simulink model "Zero_6C_5000"  (R2019a)
settings: Solver=VariableStepAuto  StartTime=0.0  StopTime=100000  RelTol=1e-3
libraries: fl_lib x40, nesl_utility x14, ee_lib x8, SimscapeFluids_lib x2, simulink x1
settings Model: Creator=Abd  LastModifiedBy=User

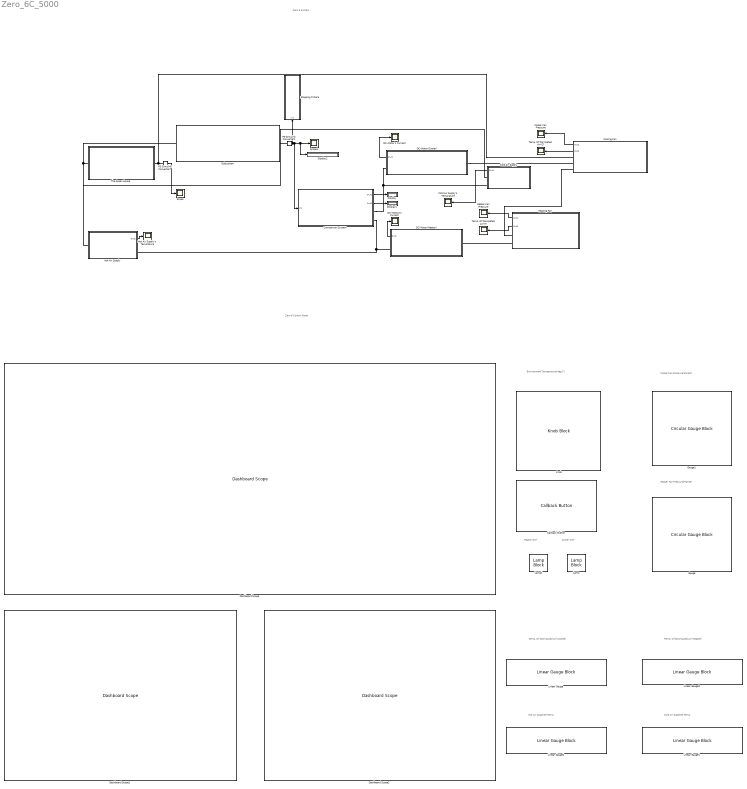
== system Zero_6C_5000 ==
  note: Environment Temperature(deg C)
  note: Temp. Of Distriputed Air(Cooled)
  note: Zero 6 System
  note: Heater ON?
  note: Cooler ON?
  note: Cooler Fan Pressure(Pa*e3)
  note: Heater Fan Pressure(Pa*e3)
  note: Temp. Of Distriputed Air(Heated)
  note: Hot Air Supplied Temp.
  note: Cold Air Supplied Temp.
  note: Zero 6 Control Panel
  Callback Button : CallbackButton  ButtonText=Start Simulation
      settings: ClickFcn=|
      | % name of your model
      | modelName = 'Zero_6C_5000';
      | 
      | % sim will simulate the model in argument
      | sim(modelName);
  Cold Air Supply : Subsystem
  Cold Air Supply's Temprature : Scope
  Comparison System : Subsystem
  Cooler Fan Pressure : Scope
  Cooling Fan : Subsystem
  DC-Motor's Current : Scope
  DC-Motor(Cooler) : Subsystem
  DC-Motor(Heater) : Subsystem
  DC-Motor2's Current : Scope
  Dashboard Scope : DashboardScope  Ymin=-20  Ymax=60
  Dashboard Scope1 : DashboardScope  ShowInitialText=off  TimeSpan=3  Ymin=-1  Ymax=4
  Dashboard Scope2 : DashboardScope  Ymin=0  Ymax=10
  Display : Display
  Display1 : Display
  Display2 : Display
      settings: Format=long_e
  Gauge : CircularGaugeBlock  LabelPosition=Hide  ScaleMin=60  ScaleMax=101.5
  Gauge1 : CircularGaugeBlock  LabelPosition=Hide  ScaleMin=60  ScaleMax=101.5
  Heater Fan Pressure : Scope
  Heating Fan : Subsystem
  Hot Air Supply : Subsystem
  Hot Air Supply's Temprature : Scope
  Knob : KnobBlock  LabelPosition=Hide  ScaleMin=-20  ScaleMax=60
  Lamp : LampBlock  LabelPosition=Hide
  Lamp1 : LampBlock  LabelPosition=Hide
  Linear Gauge{,1..3} (4 alike) : LinearGaugeBlock  LabelPosition=Hide  ScaleMin=-20  ScaleMax=60
  PS-Simulink Converter1 : nesl_utility/PS-Simulink Converter  PhysicalDomain=network_engine_domain  SubClassName=ps_output  LeftPortType=input  RightPortType=output  PseudoPeriodic=off  Frequencies=[]  Unit=1  AffineConversion=off
  PS-Simulink Converter7 : nesl_utility/PS-Simulink Converter  PhysicalDomain=network_engine_domain  SubClassName=ps_output  LeftPortType=input  RightPortType=output  PseudoPeriodic=off  Frequencies=[]  Unit=1  AffineConversion=off
  Scope : Scope
  Scope1 : Scope
  Stopping Critera : Subsystem
  Subsystem : Subsystem
  Temp. Of Dissipated Air(C) : Scope
  Temp. Of Dissipated Air(H) : Scope
  The Green House : Subsystem
  wires:
  PS-Simulink Converter1/1 -> Comparison System/1(In1), Display2/1, Scope1/1, Stopping Critera/1(In1)
  DC-Motor(Cooler)/1(Out1) -> DC-Motor's Current/1
  Cooling Fan/1(Out1) -> Cooler Fan Pressure/1
  Cooling Fan/2(Out2) -> Temp. Of Dissipated Air(C)/1
  Heating Fan/1(Out1) -> Heater Fan Pressure/1
  Heating Fan/2(Out2) -> Temp. Of Dissipated Air(H)/1
  DC-Motor(Heater)/1(Out1) -> DC-Motor2's Current/1
  Cold Air Supply/1(Out1) -> Cold Air Supply's Temprature/1
  Hot Air Supply/1(Out1) -> Hot Air Supply's Temprature/1
  PS-Simulink Converter7/1 -> Scope/1
  Comparison System/2(Out2) -> Display1/1
  Comparison System/1(Out1) -> Display/1
  connections:
  PS-Simulink Converter7/LConn1 -- Cooling Fan/RConn1 -- The Green House/RConn1
  The Green House/LConn1 -- Subsystem/LConn1 -- Cold Air Supply/RConn1 -- Hot Air Supply/LConn1
  DC-Motor(Cooler)/LConn1 -- Cooling Fan/RConn2
  Cooling Fan/RConn3 -- Heating Fan/RConn1
  Heating Fan/RConn2 -- DC-Motor(Heater)/LConn1
  Comparison System/RConn1 -- Cold Air Supply/RConn2 -- DC-Motor(Cooler)/RConn1
  Comparison System/RConn2 -- Hot Air Supply/RConn1 -- DC-Motor(Heater)/RConn1
  PS-Simulink Converter1/LConn1 -- Subsystem/RConn1

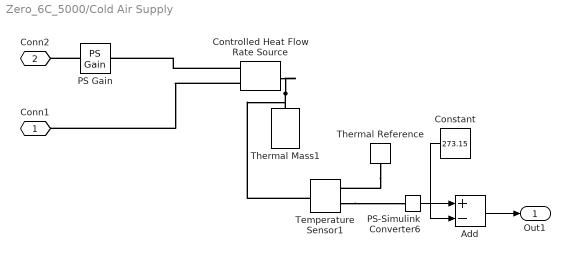
== system Zero_6C_5000/Cold Air Supply ==
  Add : Sum  Inputs=+-
  Constant : Constant  Value=273.15
  Controlled Heat Flow Rate Source : fl_lib/Thermal/Thermal Sources/Controlled Heat Flow Rate Source
      settings: SourceProductName=Simscape
  PS Gain : fl_lib/Physical Signals/Functions/PS Gain  gain=10
  PS-Simulink Converter6 : nesl_utility/PS-Simulink Converter  PhysicalDomain=network_engine_domain  SubClassName=ps_output  LeftPortType=input  RightPortType=output  PseudoPeriodic=off  Frequencies=[]  Unit=1  AffineConversion=off
  Temperature Sensor1 : fl_lib/Thermal/Thermal Sensors/Temperature Sensor
  Thermal Mass1 : fl_lib/Thermal/Thermal Elements/Thermal Mass  mass=100 kg  sp_heat=1.0045e3 J/kg/K  T_specify=on  T_priority=High  T=273.15 K  T_nominal_specify=off  T_nominal_unit=K  T_nominal_value=1  Q_specify=off  Q_priority=None  Q=0 W  Q_nominal_specify=off  Q_nominal_unit=W  Q_nominal_value=1
  Thermal Reference : fl_lib/Thermal/Thermal Elements/Thermal Reference
  Conn1 : PMIOPort  Side=Right
  Conn2 : PMIOPort  Port=2  Side=Right
  Out1 : Outport
  wires:
  Constant/1 -> Add/2
  Add/1 -> Out1/1
  PS-Simulink Converter6/1 -> Add/1
  connections:
  Temperature Sensor1/RConn2 -- PS-Simulink Converter6/LConn1
  Thermal Reference/LConn1 -- Temperature Sensor1/RConn1
  PS Gain/LConn1 -- Conn2/RConn1
  Controlled Heat Flow Rate Source/RConn2 -- Conn1/RConn1
  Thermal Mass1/LConn1 -- Controlled Heat Flow Rate Source/LConn1 -- Temperature Sensor1/LConn1
  Controlled Heat Flow Rate Source/RConn1 -- PS Gain/RConn1

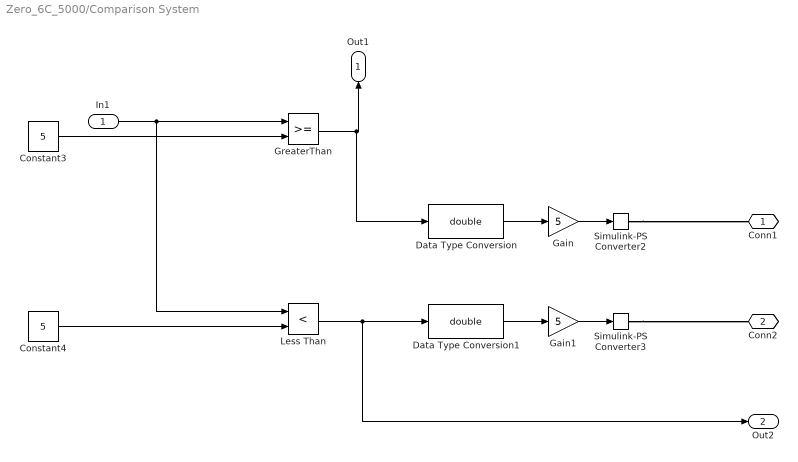
== system Zero_6C_5000/Comparison System ==
  In1 : Inport
  Constant3 : Constant  Value=5
  Constant4 : Constant  Value=5
  Data Type Conversion : DataTypeConversion  OutDataTypeStr=double
  Data Type Conversion1 : DataTypeConversion  OutDataTypeStr=double
  Gain : Gain  Gain=5
  Gain1 : Gain  Gain=5
  GreaterThan : RelationalOperator  OutDataTypeStr=boolean  RndMeth=Simplest
  Less Than : RelationalOperator  Operator=<  OutDataTypeStr=boolean  RndMeth=Simplest
  Simulink-PS Converter2 : nesl_utility/Simulink-PS Converter  PhysicalDomain=network_engine_domain  SubClassName=ps_input  LeftPortType=input  RightPortType=output  PseudoPeriodic=off  Frequencies=[]  NoiseDistribution=none  NoiseParameters=[]  Unit=1  AffineConversion=off  FilteringAndDerivatives=provide  SimscapeFilterOrder=1  InputFilterTimeConstant=0.001  UdotUserProvided=0
  Simulink-PS Converter3 : nesl_utility/Simulink-PS Converter  PhysicalDomain=network_engine_domain  SubClassName=ps_input  LeftPortType=input  RightPortType=output  PseudoPeriodic=off  Frequencies=[]  NoiseDistribution=none  NoiseParameters=[]  Unit=1  AffineConversion=off  FilteringAndDerivatives=provide  SimscapeFilterOrder=1  InputFilterTimeConstant=0.001  UdotUserProvided=0
  Conn1 : PMIOPort  Side=Right
  Conn2 : PMIOPort  Port=2  Side=Right
  Out1 : Outport
  Out2 : Outport  Port=2
  wires:
  Less Than/1 -> Out2/1, Data Type Conversion1/1
  Gain/1 -> Simulink-PS Converter2/1
  Data Type Conversion/1 -> Gain/1
  Constant3/1 -> GreaterThan/2
  Gain1/1 -> Simulink-PS Converter3/1
  GreaterThan/1 -> Data Type Conversion/1, Out1/1
  Constant4/1 -> Less Than/2
  Data Type Conversion1/1 -> Gain1/1
  In1/1 -> GreaterThan/1, Less Than/1
  connections:
  Simulink-PS Converter3/RConn1 -- Conn2/RConn1
  Simulink-PS Converter2/RConn1 -- Conn1/RConn1

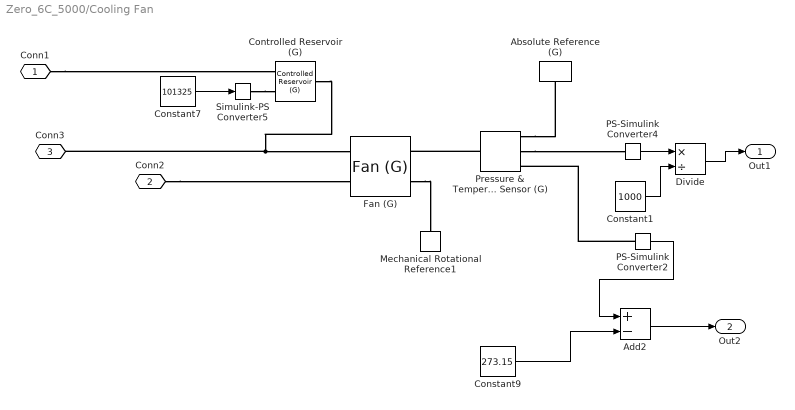
== system Zero_6C_5000/Cooling Fan ==
  Absolute Reference (G) : fl_lib/Gas/Elements/Absolute Reference (G)
      settings: SourceProductName=Simscape  SourceProductBaseCode=SS
  Add2 : Sum  Inputs=+-
  Constant1 : Constant  Value=1000
  Constant7 : Constant  Value=101325
  Constant9 : Constant  Value=273.15
  Controlled Reservoir (G) : fl_lib/Gas/Elements/Controlled Reservoir (G)  area_A=0.01 m^2
      settings: SourceProductName=Simscape  SourceProductBaseCode=SS
  Divide : Product  Inputs=*/
  Fan (G) : SimscapeFluids_lib/Gas/Turbomachinery/Fan (G)  fan_spec=fluids.gas.enum.fan_spec.table1D  mech_orientation=simscape.enum.posneg.positive  flow_rate_1D_TLU=[4.7, 5.2, 5.7, 6.1, 6.6] m^3/s  Dp_1D_TLU=[1120, 995.36, 870.94, 746.52, 622.1] Pa  eta_1D_TLU=[.1, .2, .25, .15, .1]  rho_ref_1D=1.2 kg/m^3  omega_ref_1D=910 rpm  omega_Dp_TLU=[450, 500, 550, 600, 650] rpm  flow_rate_Dp_TLU=[.2, .3, .4, .5] m^3/s  Dp_TLU=[675, 650, 560, 420; 830, 800, 695, 520; 1008, 966, 840, 630; 1200, 1150, 1000, 750; 1370, 1300, 1250, 1000] Pa  eta_Dp_TLU=[.22, .23, .25, .24; .38, .39, .4, .34; .58, .6, .62, .6; .81, .82, .84, .8; .88, .91, .95, .9]  omega_flow_TLU=[1800, 2000, 2400, 2800, 3000] rpm  Dp_flow_TLU=[1 / 8, 1 / 4, 3 / 8, 1 / 2] * 3386.4 Pa  flow_rate_TLU=[.3282, .2965, .2556, .1973; .8254, .71, .5876, .4545; 1.2018, 1.0829, .9083, .7034; 1.5065, 1.4098, 1.2722, .9844; 1.8368, 1.7507, 1.6055, 1.2417] m^3/s  eta_flow_TLU=[.22, .23, .25, .24; .38, .39, .4, .34; .58, .6, .62, .6; .81, .82, .84, .8; .88, .91, .95, .9]  omega_DpMax_TLU=[1800, 2000, 2400, 2800, 3000] rpm  DpMax_TLU=[1 / 8, 1 / 4, 3 / 8, 1 / 2, 5 / 8] * 3386.4 Pa  omega_flow_TLU_=[1800, 2000, 2400, 2800, 3000] rpm  Dp_DpMax_TLU=linspace(0, 1, 7)  flow_rate_TLU_=[.3282, .2965, .2556, .1973, .1799, .1288, .0736; .8254, .71, .5876, .4545, .4157, .2967, .1696; 1.2018, 1.0829, .9083, .7034, .6415, .4584, .2619; 1.5065, 1.4098, 1.2722, .9844, .8991, .6418, .3668; 1.8368, 1.7507, 1.6055, 1.2417, 1.1337, .8098, .464] m^3/s  eta_flow_TLU_=[.22, .23, .25, .26, .27, .275, .28; .38, .39, .4, .41, .42, .425, .43; .48, .5, .52, .54, .55, .54, .53; .4, .42, .44, .46, .48, .45, .44; .42, .43, .45, .47, .49, .46, .44]  rho_ref_2D=1.2 kg/m^3  omega_threshold=1 rpm  area_A=0.01 m^2  area_B=0.01 m^2
      settings: SourceProductName=Simscape Fluids  SourceProductBaseCode=SH
  Mechanical Rotational Reference1 : fl_lib/Mechanical/Rotational Elements/Mechanical Rotational Reference
  PS-Simulink Converter2 : nesl_utility/PS-Simulink Converter  PhysicalDomain=network_engine_domain  SubClassName=ps_output  LeftPortType=input  RightPortType=output  PseudoPeriodic=off  Frequencies=[]  Unit=1  AffineConversion=off
  PS-Simulink Converter4 : nesl_utility/PS-Simulink Converter  PhysicalDomain=network_engine_domain  SubClassName=ps_output  LeftPortType=input  RightPortType=output  PseudoPeriodic=off  Frequencies=[]  Unit=1  AffineConversion=off
  Pressure & Temperature Sensor (G) : fl_lib/Gas/Sensors/Pressure & Temperature Sensor (G)
      settings: SourceProductName=Simscape  SourceProductBaseCode=SS
  Simulink-PS Converter5 : nesl_utility/Simulink-PS Converter  PhysicalDomain=network_engine_domain  SubClassName=ps_input  LeftPortType=input  RightPortType=output  PseudoPeriodic=off  Frequencies=[]  NoiseDistribution=none  NoiseParameters=[]  Unit=1  AffineConversion=off  FilteringAndDerivatives=provide  SimscapeFilterOrder=1  InputFilterTimeConstant=0.001  UdotUserProvided=0
  Conn1 : PMIOPort  Side=Right
  Conn2 : PMIOPort  Port=2  Side=Right
  Conn3 : PMIOPort  Port=3  Side=Right
  Out1 : Outport
  Out2 : Outport  Port=2
  wires:
  Constant9/1 -> Add2/2
  Constant7/1 -> Simulink-PS Converter5/1
  PS-Simulink Converter2/1 -> Add2/1
  Add2/1 -> Out2/1
  Divide/1 -> Out1/1
  PS-Simulink Converter4/1 -> Divide/1
  Constant1/1 -> Divide/2
  connections:
  Controlled Reservoir (G)/LConn1 -- Fan (G)/RConn1 -- Conn3/RConn1
  Pressure & Temperature Sensor (G)/RConn2 -- PS-Simulink Converter4/LConn1
  PS-Simulink Converter2/LConn1 -- Pressure & Temperature Sensor (G)/RConn3
  Pressure & Temperature Sensor (G)/RConn1 -- Absolute Reference (G)/LConn1
  Simulink-PS Converter5/RConn1 -- Controlled Reservoir (G)/RConn2
  Conn1/RConn1 -- Controlled Reservoir (G)/RConn1
  Pressure & Temperature Sensor (G)/LConn1 -- Fan (G)/LConn1
  Fan (G)/LConn2 -- Mechanical Rotational Reference1/LConn1
  Conn2/RConn1 -- Fan (G)/RConn2

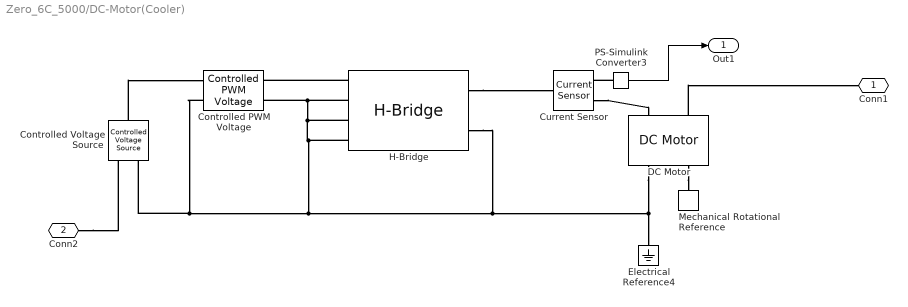
== system Zero_6C_5000/DC-Motor(Cooler) ==
  Controlled PWM Voltage : ee_lib/Integrated Circuits/Controlled PWM Voltage  F=4000 Hz  TD=0 s  pulse_width_offset=0 s  pulse_min=0 s  Vmin=0 V  Vmax=5 V  Vm=5 V  pwm_or_av=2  event_type=1  sample_time=1e-6 s  u_min=0  u_max=1
      settings: SourceProductName=Simscape Electrical
  Controlled Voltage Source : fl_lib/Electrical/Electrical Sources/Controlled Voltage Source
  Current Sensor : fl_lib/Electrical/Electrical Sensors/Current Sensor
  DC Motor : ee_lib/Electromechanical/Brushed Motors/DC Motor  parameterization=3  Ra=3.9 Ohm  La=0.01 H  emf_or_torque=1  Kv=0.072e-3 V/rpm  Ki=6.876e-4 N*m/A  T_stall=0.24e-3 N*m  w_max=4000 rpm  w_rated=2500 rpm  P_rated=10 W  V_rated=12 V  J=2000 g*cm^2  lam_param=1  lam=1e-6 N*m/(rad/s)  i_noload=0 A  V_i_noload=1.5 V  speed0=0 rpm  alpha=3.93e-3 1/K  Tmeas=25 degC  thermal_mass=100 J/K  initial_temperature=25 degC
      settings: SourceProductName=Simscape Electrical
  Electrical Reference4 : fl_lib/Electrical/Electrical Elements/Electrical Reference
  H-Bridge : ee_lib/Semiconductors & Converters/Converters/H-Bridge  Venable=2.5 V  Vmax=5.0 V  Vreverse=2.5 V  Vbrake=2.5 V  Vm=12 V  pwm_or_av=2  discontinuous=0  freewheeling_mode=1  freewheeling_mode_disc=1  Ron=0.1 Ohm  Don=0.05 Ohm  Rload=10 Ohm  Lload=1e-5 H  F=10 kHz  thermal_mass=100 J/K  initial_temperature=298.15 K  Ron2=0.1 Ohm  Don2=0.05 Ohm  Tmeas=298.15 K  Tmeas2=398.15 K
      settings: SourceProductName=Simscape Electrical
  Mechanical Rotational Reference : fl_lib/Mechanical/Rotational Elements/Mechanical Rotational Reference
  PS-Simulink Converter3 : nesl_utility/PS-Simulink Converter  PhysicalDomain=network_engine_domain  SubClassName=ps_output  LeftPortType=input  RightPortType=output  PseudoPeriodic=off  Frequencies=[]  Unit=1  AffineConversion=off
  Conn1 : PMIOPort  Side=Left
  Conn2 : PMIOPort  Port=2  Side=Right
  Out1 : Outport
  wires:
  PS-Simulink Converter3/1 -> Out1/1
  connections:
  H-Bridge/LConn3 -- Electrical Reference4/LConn1 -- DC Motor/RConn1 -- H-Bridge/RConn2 -- Controlled Voltage Source/RConn2 -- Controlled PWM Voltage/LConn2 -- H-Bridge/LConn4 -- H-Bridge/LConn2 -- Controlled PWM Voltage/RConn2
  Controlled Voltage Source/LConn1 -- Controlled PWM Voltage/LConn1
  DC Motor/RConn2 -- Mechanical Rotational Reference/LConn1
  DC Motor/LConn2 -- Conn1/RConn1
  H-Bridge/LConn1 -- Controlled PWM Voltage/RConn1
  PS-Simulink Converter3/LConn1 -- Current Sensor/RConn1
  Current Sensor/RConn2 -- DC Motor/LConn1
  H-Bridge/RConn1 -- Current Sensor/LConn1
  Conn2/RConn1 -- Controlled Voltage Source/RConn1

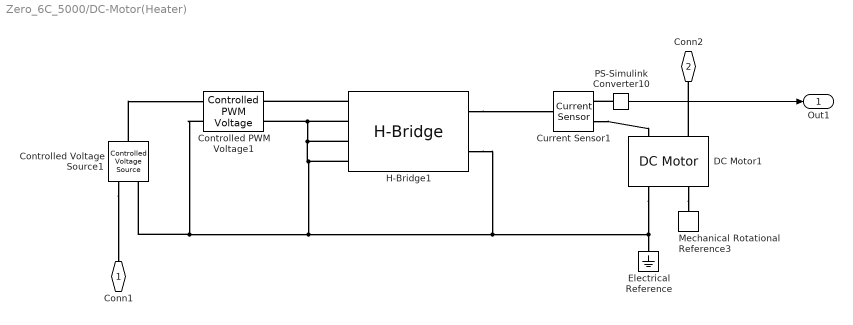
== system Zero_6C_5000/DC-Motor(Heater) ==
  Controlled PWM Voltage1 : ee_lib/Integrated Circuits/Controlled PWM Voltage  F=4000 Hz  TD=0 s  pulse_width_offset=0 s  pulse_min=0 s  Vmin=0 V  Vmax=5 V  Vm=5 V  pwm_or_av=2  event_type=1  sample_time=1e-6 s  u_min=0  u_max=1
      settings: SourceProductName=Simscape Electrical
  Controlled Voltage Source1 : fl_lib/Electrical/Electrical Sources/Controlled Voltage Source
  Current Sensor1 : fl_lib/Electrical/Electrical Sensors/Current Sensor
  DC Motor1 : ee_lib/Electromechanical/Brushed Motors/DC Motor  parameterization=3  Ra=3.9 Ohm  La=0.01 H  emf_or_torque=1  Kv=0.072e-3 V/rpm  Ki=6.876e-4 N*m/A  T_stall=0.24e-3 N*m  w_max=4000 rpm  w_rated=2500 rpm  P_rated=10 W  V_rated=12 V  J=2000 g*cm^2  lam_param=1  lam=1e-6 N*m/(rad/s)  i_noload=0 A  V_i_noload=1.5 V  speed0=0 rpm  alpha=3.93e-3 1/K  Tmeas=25 degC  thermal_mass=100 J/K  initial_temperature=25 degC
      settings: SourceProductName=Simscape Electrical
  Electrical Reference : fl_lib/Electrical/Electrical Elements/Electrical Reference
  H-Bridge1 : ee_lib/Semiconductors & Converters/Converters/H-Bridge  Venable=2.5 V  Vmax=5.0 V  Vreverse=2.5 V  Vbrake=2.5 V  Vm=12 V  pwm_or_av=2  discontinuous=0  freewheeling_mode=1  freewheeling_mode_disc=1  Ron=0.1 Ohm  Don=0.05 Ohm  Rload=10 Ohm  Lload=1e-5 H  F=10 kHz  thermal_mass=100 J/K  initial_temperature=298.15 K  Ron2=0.1 Ohm  Don2=0.05 Ohm  Tmeas=298.15 K  Tmeas2=398.15 K
      settings: SourceProductName=Simscape Electrical
  Mechanical Rotational Reference3 : fl_lib/Mechanical/Rotational Elements/Mechanical Rotational Reference
  PS-Simulink Converter10 : nesl_utility/PS-Simulink Converter  PhysicalDomain=network_engine_domain  SubClassName=ps_output  LeftPortType=input  RightPortType=output  PseudoPeriodic=off  Frequencies=[]  Unit=1  AffineConversion=off
  Conn1 : PMIOPort  Side=Right
  Conn2 : PMIOPort  Port=2  Side=Left
  Out1 : Outport
  wires:
  PS-Simulink Converter10/1 -> Out1/1
  connections:
  Controlled Voltage Source1/RConn1 -- Conn1/RConn1
  PS-Simulink Converter10/LConn1 -- Current Sensor1/RConn1
  H-Bridge1/LConn3 -- Controlled PWM Voltage1/RConn2 -- H-Bridge1/LConn2 -- H-Bridge1/LConn4 -- Controlled PWM Voltage1/LConn2 -- Controlled Voltage Source1/RConn2 -- H-Bridge1/RConn2 -- Electrical Reference/LConn1 -- DC Motor1/RConn1
  Controlled Voltage Source1/LConn1 -- Controlled PWM Voltage1/LConn1
  Current Sensor1/RConn2 -- DC Motor1/LConn1
  DC Motor1/RConn2 -- Mechanical Rotational Reference3/LConn1
  H-Bridge1/RConn1 -- Current Sensor1/LConn1
  H-Bridge1/LConn1 -- Controlled PWM Voltage1/RConn1
  DC Motor1/LConn2 -- Conn2/RConn1

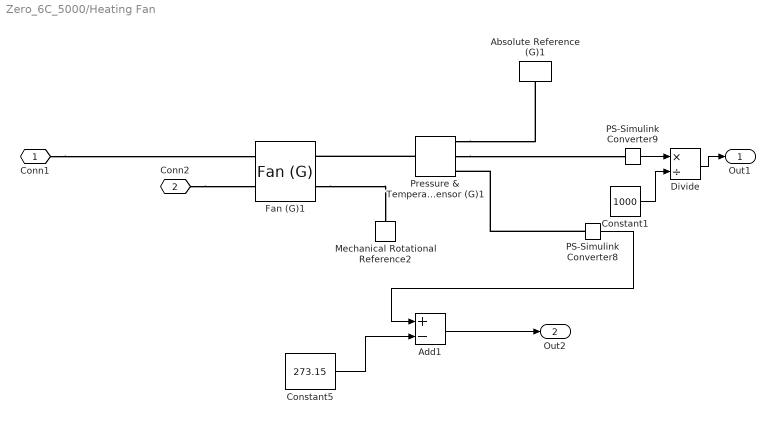
== system Zero_6C_5000/Heating Fan ==
  Absolute Reference (G)1 : fl_lib/Gas/Elements/Absolute Reference (G)
      settings: SourceProductName=Simscape  SourceProductBaseCode=SS
  Add1 : Sum  Inputs=+-
  Constant1 : Constant  Value=1000
  Constant5 : Constant  Value=273.15
  Divide : Product  Inputs=*/
  Fan (G)1 : SimscapeFluids_lib/Gas/Turbomachinery/Fan (G)  fan_spec=fluids.gas.enum.fan_spec.table1D  mech_orientation=simscape.enum.posneg.positive  flow_rate_1D_TLU=[4.7, 5.2, 5.7, 6.1, 6.6] m^3/s  Dp_1D_TLU=[1120, 995.36, 870.94, 746.52, 622.1] Pa  eta_1D_TLU=[.1, .2, .25, .15, .1]  rho_ref_1D=1.2 kg/m^3  omega_ref_1D=910 rpm  omega_Dp_TLU=[450, 500, 550, 600, 650] rpm  flow_rate_Dp_TLU=[.2, .3, .4, .5] m^3/s  Dp_TLU=[675, 650, 560, 420; 830, 800, 695, 520; 1008, 966, 840, 630; 1200, 1150, 1000, 750; 1370, 1300, 1250, 1000] Pa  eta_Dp_TLU=[.22, .23, .25, .24; .38, .39, .4, .34; .58, .6, .62, .6; .81, .82, .84, .8; .88, .91, .95, .9]  omega_flow_TLU=[1800, 2000, 2400, 2800, 3000] rpm  Dp_flow_TLU=[1 / 8, 1 / 4, 3 / 8, 1 / 2] * 3386.4 Pa  flow_rate_TLU=[.3282, .2965, .2556, .1973; .8254, .71, .5876, .4545; 1.2018, 1.0829, .9083, .7034; 1.5065, 1.4098, 1.2722, .9844; 1.8368, 1.7507, 1.6055, 1.2417] m^3/s  eta_flow_TLU=[.22, .23, .25, .24; .38, .39, .4, .34; .58, .6, .62, .6; .81, .82, .84, .8; .88, .91, .95, .9]  omega_DpMax_TLU=[1800, 2000, 2400, 2800, 3000] rpm  DpMax_TLU=[1 / 8, 1 / 4, 3 / 8, 1 / 2, 5 / 8] * 3386.4 Pa  omega_flow_TLU_=[1800, 2000, 2400, 2800, 3000] rpm  Dp_DpMax_TLU=linspace(0, 1, 7)  flow_rate_TLU_=[.3282, .2965, .2556, .1973, .1799, .1288, .0736; .8254, .71, .5876, .4545, .4157, .2967, .1696; 1.2018, 1.0829, .9083, .7034, .6415, .4584, .2619; 1.5065, 1.4098, 1.2722, .9844, .8991, .6418, .3668; 1.8368, 1.7507, 1.6055, 1.2417, 1.1337, .8098, .464] m^3/s  eta_flow_TLU_=[.22, .23, .25, .26, .27, .275, .28; .38, .39, .4, .41, .42, .425, .43; .48, .5, .52, .54, .55, .54, .53; .4, .42, .44, .46, .48, .45, .44; .42, .43, .45, .47, .49, .46, .44]  rho_ref_2D=1.2 kg/m^3  omega_threshold=1 rpm  area_A=0.01 m^2  area_B=0.01 m^2
      settings: SourceProductName=Simscape Fluids  SourceProductBaseCode=SH
  Mechanical Rotational Reference2 : fl_lib/Mechanical/Rotational Elements/Mechanical Rotational Reference
  PS-Simulink Converter8 : nesl_utility/PS-Simulink Converter  PhysicalDomain=network_engine_domain  SubClassName=ps_output  LeftPortType=input  RightPortType=output  PseudoPeriodic=off  Frequencies=[]  Unit=1  AffineConversion=off
  PS-Simulink Converter9 : nesl_utility/PS-Simulink Converter  PhysicalDomain=network_engine_domain  SubClassName=ps_output  LeftPortType=input  RightPortType=output  PseudoPeriodic=off  Frequencies=[]  Unit=1  AffineConversion=off
  Pressure & Temperature Sensor (G)1 : fl_lib/Gas/Sensors/Pressure & Temperature Sensor (G)
      settings: SourceProductName=Simscape  SourceProductBaseCode=SS
  Conn1 : PMIOPort  Side=Right
  Conn2 : PMIOPort  Port=2  Side=Right
  Out1 : Outport
  Out2 : Outport  Port=2
  wires:
  PS-Simulink Converter8/1 -> Add1/1
  Add1/1 -> Out2/1
  Constant5/1 -> Add1/2
  PS-Simulink Converter9/1 -> Divide/1
  Constant1/1 -> Divide/2
  Divide/1 -> Out1/1
  connections:
  PS-Simulink Converter8/LConn1 -- Pressure & Temperature Sensor (G)1/RConn3
  Pressure & Temperature Sensor (G)1/RConn2 -- PS-Simulink Converter9/LConn1
  Pressure & Temperature Sensor (G)1/LConn1 -- Fan (G)1/LConn1
  Conn2/RConn1 -- Fan (G)1/RConn2
  Fan (G)1/LConn2 -- Mechanical Rotational Reference2/LConn1
  Pressure & Temperature Sensor (G)1/RConn1 -- Absolute Reference (G)1/LConn1
  Conn1/RConn1 -- Fan (G)1/RConn1

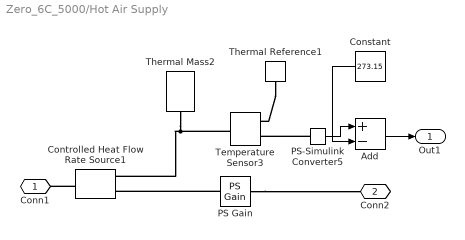
== system Zero_6C_5000/Hot Air Supply ==
  Add : Sum  Inputs=+-
  Constant : Constant  Value=273.15
  Controlled Heat Flow Rate Source1 : fl_lib/Thermal/Thermal Sources/Controlled Heat Flow Rate Source
      settings: SourceProductName=Simscape
  PS Gain : fl_lib/Physical Signals/Functions/PS Gain  gain=10
  PS-Simulink Converter5 : nesl_utility/PS-Simulink Converter  PhysicalDomain=network_engine_domain  SubClassName=ps_output  LeftPortType=input  RightPortType=output  PseudoPeriodic=off  Frequencies=[]  Unit=1  AffineConversion=off
  Temperature Sensor3 : fl_lib/Thermal/Thermal Sensors/Temperature Sensor
  Thermal Mass2 : fl_lib/Thermal/Thermal Elements/Thermal Mass  mass=100 kg  sp_heat=1.0045e+3 J/kg/K  T_specify=on  T_priority=High  T=273.15+40 K  T_nominal_specify=off  T_nominal_unit=K  T_nominal_value=1  Q_specify=off  Q_priority=None  Q=0 W  Q_nominal_specify=off  Q_nominal_unit=W  Q_nominal_value=1
  Thermal Reference1 : fl_lib/Thermal/Thermal Elements/Thermal Reference
  Conn1 : PMIOPort  Side=Left
  Conn2 : PMIOPort  Port=2  Side=Right
  Out1 : Outport
  wires:
  Add/1 -> Out1/1
  PS-Simulink Converter5/1 -> Add/1
  Constant/1 -> Add/2
  connections:
  PS-Simulink Converter5/LConn1 -- Temperature Sensor3/RConn2
  Controlled Heat Flow Rate Source1/LConn1 -- Conn1/RConn1
  Thermal Mass2/LConn1 -- Controlled Heat Flow Rate Source1/RConn2 -- Temperature Sensor3/LConn1
  Thermal Reference1/LConn1 -- Temperature Sensor3/RConn1
  PS Gain/LConn1 -- Conn2/RConn1
  PS Gain/RConn1 -- Controlled Heat Flow Rate Source1/RConn1

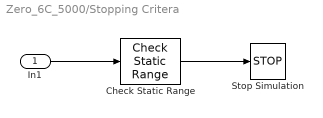
== system Zero_6C_5000/Stopping Critera ==
  In1 : Inport
  Check Static Range : simulink/Model Verification/Check  Static Range  Description=4.999995 <= u <= 5.000005  max=5.000005  max_included=on  min=4.999995  min_included=on  enabled=off  stopWhenAssertionFail=on  export=on  icon=graphic
      settings: SourceProductName=Simulink  SourceProductBaseCode=SL
  Stop Simulation : Stop
  wires:
  In1/1 -> Check Static Range/1
  Check Static Range/1 -> Stop Simulation/1

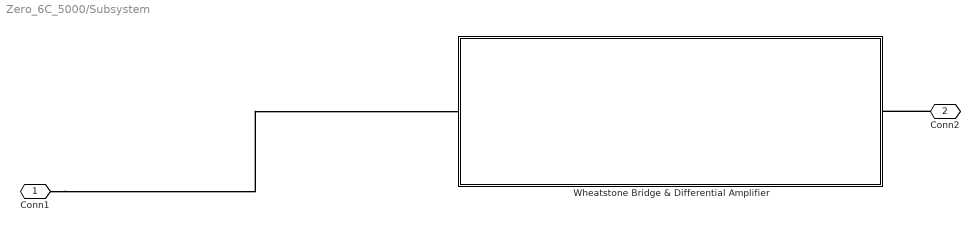
== system Zero_6C_5000/Subsystem ==
  Wheatstone Bridge & Differential Amplifier : Subsystem
  Conn1 : PMIOPort  Side=Left
  Conn2 : PMIOPort  Port=2  Side=Right
  connections:
  Conn2/RConn1 -- Wheatstone Bridge & Differential Amplifier/RConn1
  Conn1/RConn1 -- Wheatstone Bridge & Differential Amplifier/LConn1

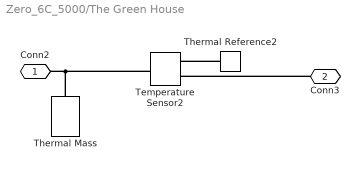
== system Zero_6C_5000/The Green House ==
  Temperature Sensor2 : fl_lib/Thermal/Thermal Sensors/Temperature Sensor
  Thermal Mass : fl_lib/Thermal/Thermal Elements/Thermal Mass  mass=100 kg  sp_heat=1.0045e3 J/kg/K  T_specify=on  T_priority=High  T=300 degC  T_nominal_specify=off  T_nominal_unit=K  T_nominal_value=1  Q_specify=off  Q_priority=None  Q=0 W  Q_nominal_specify=off  Q_nominal_unit=W  Q_nominal_value=1
  Thermal Reference2 : fl_lib/Thermal/Thermal Elements/Thermal Reference
  Conn2 : PMIOPort  Side=Left
  Conn3 : PMIOPort  Port=2  Side=Right
  connections:
  Temperature Sensor2/LConn1 -- Thermal Mass/LConn1 -- Conn2/RConn1
  Thermal Reference2/LConn1 -- Temperature Sensor2/RConn1
  Conn3/RConn1 -- Temperature Sensor2/RConn2

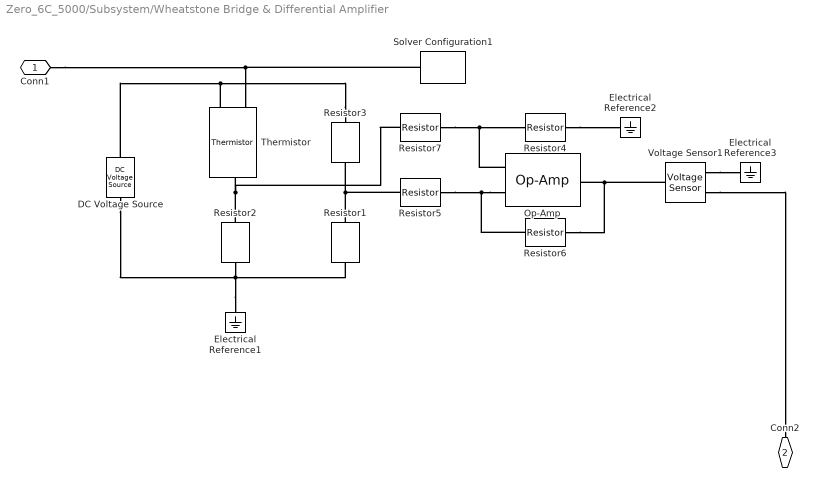
== system Zero_6C_5000/Subsystem/Wheatstone Bridge & Differential Amplifier ==
  DC Voltage Source : ee_lib/Additional Components/SPICE Sources/DC Voltage Source  DC=10 V
      settings: SourceProductName=Simscape Electrical
  Electrical Reference1 : fl_lib/Electrical/Electrical Elements/Electrical Reference
  Electrical Reference2 : fl_lib/Electrical/Electrical Elements/Electrical Reference
  Electrical Reference3 : fl_lib/Electrical/Electrical Elements/Electrical Reference
  Op-Amp : fl_lib/Electrical/Electrical Elements/Op-Amp  outI_specify=off  outI_priority=None  outI=0 A  outI_nominal_specify=off  outI_nominal_unit=A  outI_nominal_value=1
  Resistor1 : fl_lib/Electrical/Electrical Elements/Resistor  R="2.928279149950059  kOhm"  i_specify=off  i_priority=None  i=0 A  i_nominal_specify=off  i_nominal_unit=A  i_nominal_value=1  v_specify=off  v_priority=None  v=0 V  v_nominal_specify=off  v_nominal_unit=V  v_nominal_value=1
  Resistor2 : fl_lib/Electrical/Electrical Elements/Resistor  R="2.928279149950059  kOhm"  i_specify=off  i_priority=None  i=0 A  i_nominal_specify=off  i_nominal_unit=A  i_nominal_value=1  v_specify=off  v_priority=None  v=0 V  v_nominal_specify=off  v_nominal_unit=V  v_nominal_value=1
  Resistor3 : fl_lib/Electrical/Electrical Elements/Resistor  R="2.928279149950059  kOhm"  i_specify=off  i_priority=None  i=0 A  i_nominal_specify=off  i_nominal_unit=A  i_nominal_value=1  v_specify=off  v_priority=None  v=0 V  v_nominal_specify=off  v_nominal_unit=V  v_nominal_value=1
  Resistor4 : fl_lib/Electrical/Electrical Elements/Resistor  R=2.339446759459657 kOhm  i_specify=off  i_priority=None  i=0 A  i_nominal_specify=off  i_nominal_unit=A  i_nominal_value=1  v_specify=off  v_priority=None  v=0 V  v_nominal_specify=off  v_nominal_unit=V  v_nominal_value=1
  Resistor5 : fl_lib/Electrical/Electrical Elements/Resistor  R=100 Ohm  i_specify=off  i_priority=None  i=0 A  i_nominal_specify=off  i_nominal_unit=A  i_nominal_value=1  v_specify=off  v_priority=None  v=0 V  v_nominal_specify=off  v_nominal_unit=V  v_nominal_value=1
  Resistor6 : fl_lib/Electrical/Electrical Elements/Resistor  R=2.339446759459657 kOhm  i_specify=off  i_priority=None  i=0 A  i_nominal_specify=off  i_nominal_unit=A  i_nominal_value=1  v_specify=off  v_priority=None  v=0 V  v_nominal_specify=off  v_nominal_unit=V  v_nominal_value=1
  Resistor7 : fl_lib/Electrical/Electrical Elements/Resistor  R=100 Ohm  i_specify=off  i_priority=None  i=0 A  i_nominal_specify=off  i_nominal_unit=A  i_nominal_value=1  v_specify=off  v_priority=None  v=0 V  v_nominal_specify=off  v_nominal_unit=V  v_nominal_value=1
  Solver Configuration1 : nesl_utility/Solver Configuration  PhysicalDomain=network_engine_domain  SubClassName=solver  LeftPortType=input  RightPortType=generic  Tones=[]  Harmonics=[]  SimulateNoise=off  Profile=off  UseLocalSampling=off  EnableSwitchedLinearOptims=on  FrequencyDomain=off  UseCCode=off  RelTol=0.001  AbsTol=1e-06  MinStep=1e-09  ToWorkspace=off  RevertToSquareIcSolve=off  NumHomotopyIterations=100  PhasorMode=off  PhasorModeNumHarmonics=1  DoDC=off  ResidualTolerance=1e-09  UseLocalSolver=off  LocalSolverChoice=NE_BACKWARD_EULER_ADVANCER  LocalSolverSampleTime=0.001  DoFixedCost=off  MaxNonlinIter=3  MaxModeIter=2  LinearAlgebra=auto  EquationFormulation=NE_TIME_EF  DelaysMemoryBudget=1024  AutomaticFiltering=on  FilteringTimeConstant=0.001  PartitionStorageMethod=AS_NEEDED  PartitionMemoryBudget=1024  PartitionMethod=ROBUST
  Thermistor : ee_lib/Sensors & Transducers/Thermistor  R0=1000 Ohm  Bparam=3500 K  T0=298.15 K  tc=5.0 s  K_d=0.75e-3 W/K  T_specify=off  T_priority=High  T=298.15 K  T_nominal_specify=off  T_nominal_unit=K  T_nominal_value=1
      settings: SourceProductName=Simscape Electrical  SourceProductBaseCode=PS
  Voltage Sensor1 : fl_lib/Electrical/Electrical Sensors/Voltage Sensor
  Conn1 : PMIOPort  Side=Left
  Conn2 : PMIOPort  Port=2  Side=Right
  connections:
  Resistor1/LConn1 -- Resistor3/RConn1 -- Resistor5/LConn1
  Op-Amp/LConn2 -- Resistor6/LConn1 -- Resistor5/RConn1
  Thermistor/RConn1 -- Resistor2/LConn1 -- Resistor7/LConn1
  Resistor3/LConn1 -- Thermistor/LConn2 -- DC Voltage Source/LConn1
  Electrical Reference1/LConn1 -- Resistor2/RConn1 -- DC Voltage Source/RConn1 -- Resistor1/RConn1
  Op-Amp/RConn1 -- Resistor6/RConn1 -- Voltage Sensor1/LConn1
  Op-Amp/LConn1 -- Resistor4/LConn1 -- Resistor7/RConn1
  Voltage Sensor1/RConn2 -- Electrical Reference3/LConn1
  Solver Configuration1/RConn1 -- Conn1/RConn1 -- Thermistor/LConn1
  Resistor4/RConn1 -- Electrical Reference2/LConn1
  Voltage Sensor1/RConn1 -- Conn2/RConn1
